simulink model "sim_2_3_matlab2024"  (R2024b)
settings: Solver=ode4  StartTime=0.0  StopTime=T_SIM  FixedStep=1e-3  RelTol=1e-3
values from neighbouring files (symbols this model uses):
  kf = 10    [EX_opt_2_leo.m]    (also in part2.m = 1; script_2_motion_planning.m)
  ki = 14    [EX_opt_2_leo.m]    (also in part2.m = 10; script_2_motion_planning.m = 4.5)
  qf = [1; 1; pi/2]    [EX_opt_2_leo.m]    (also in part2.m = [xf;yf;thetaf]; script_2_motion_planning.m)
  qi = [-1; -1; pi/2]    [EX_opt_2_leo.m]    (also in part2.m = [xi;yi;thetai]; script_2_motion_planning.m)
  Ta = 1    [fcn.m]    (also in part2.m = 2)
  Tc = 2    [fcn.m]    (also in part2.m = 3)
settings Model: Creator=alber  LastModifiedBy=loren
settings RTWCC: GPUComputeCapability=3.5

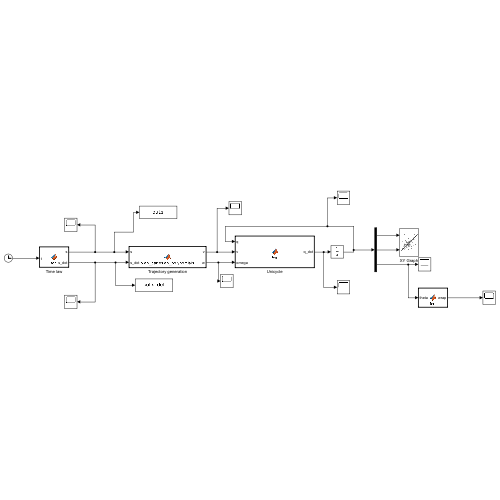
[thumbnail: Simulink's stored preview of the top-level diagram]
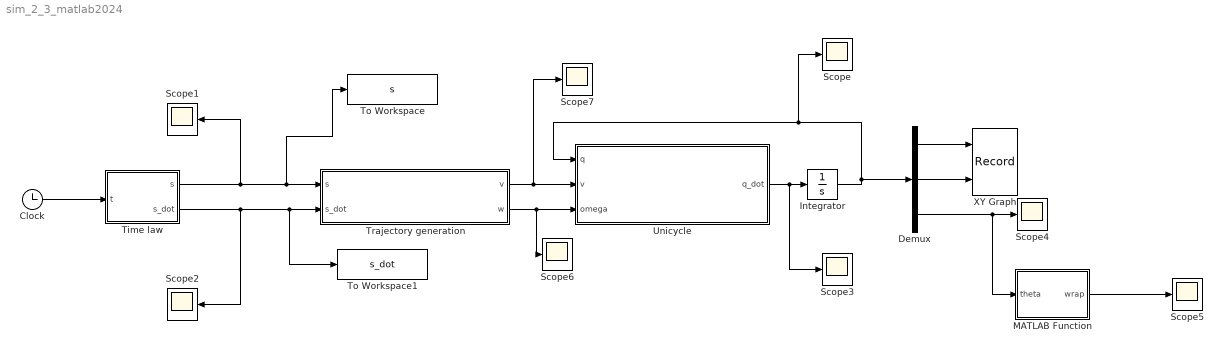
== system sim_2_3_matlab2024 ==
  Clock : Clock
  Demux : Demux  Outputs=3
  Integrator : Integrator  InitialCondition=qi
  MATLAB Function : MATLAB Function  TreatAsAtomicUnit=on
  Scope{,1..7} (8 alike) : Scope
  Time law : MATLAB Function  TreatAsAtomicUnit=on
  To Workspace : ToWorkspace  VariableName=s  SaveFormat=Timeseries  SampleTime=-1
  To Workspace1 : ToWorkspace  VariableName=s_dot  SaveFormat=Timeseries  SampleTime=-1
  Trajectory generation : MATLAB Function  TreatAsAtomicUnit=on
  Unicycle : MATLAB Function  TreatAsAtomicUnit=on
  XY Graph : Record  FileSettingsInternal="{\"entries\":[{\"content\":{\"excelSettings\":{\"content\":{},\"type\":\"Streamout.ExcelSettings\"}},\"type\":\"Streamout.FileSettingStorage\",\"uuid\":\"\"}],\"packageUris\":[\"http:\\/\\/schema.mathworks.com\\/mf0\\/streamout_blocks\\/R2020a\"],\"version\":\"1.0\"}"  Layout=[1 1]  SignalsInternal="{\"entries\":[{\"content\":{\"signals\":[{\"content\":{\"blockPath\":[],\"dimensions\":[1,1],\"domain\":\"\",\"lineColor\":\"#a2142f\",\"plots\":[ 1 ],\"port\":1,\"sid\":[\"\"],\"signalID\":1,\"signalName\":\"Demux:1\"},\"type\":\"RecordBlkView.Signal\",\"uuid\":\"\"},{\"content\":{\"blockPath\":[],\"dimensions\":[1,1],\"domain\":\"\",\"lineColor\":\"#139fff\",\"plots\":[ 1 ],\"port\":2,\"sid\":[\"\"],\"signalID\":2,\"signalName\":\"Demux:2\"},\"type\":\"RecordBlkView.Signal\",\"uuid\":\"\"}]},\"type\":\"RecordBlkView.InputSignals\",\"uuid\":\"\"}],\"packageUris\":[\"http:\\/\\/schema.mathworks.com\\/mf0\\/streamout_blocks\\/R2020a\"],\"version\":\"1.0\"}"  VisualizationBindings="{\"xyplotplugin\":{\"info\":[{\"series\":[{\"bindingParametersList\":[{\"parameter\":\"X-Axis\",\"signalID\":1,\"signalName\":\"Demux:1\"},{\"parameter\":\"Y-Axis\",\"signalID\":2,\"signalName\":\"Demux:2\"}],\"seriesID\":0}],\"subplotID\":1}]}}"  CompatibilityTag=XY
  wires:
  Clock/1 -> Time law/1(t)
  Time law/1(s) -> Scope1/1, To Workspace/1, Trajectory generation/1(s)
  Time law/2(s_dot) -> Scope2/1, To Workspace1/1, Trajectory generation/2(s_dot)
  Trajectory generation/1(v) -> Scope7/1, Unicycle/2(v)
  Trajectory generation/2(w) -> Scope6/1, Unicycle/3(omega)
  Unicycle/1(q_dot) -> Scope3/1, Integrator/1
  Demux/1 -> XY Graph/1
  Integrator/1 -> Scope/1, Unicycle/1(q), Demux/1
  MATLAB Function/1(wrap) -> Scope5/1
  Demux/2 -> XY Graph/2
  Demux/3 -> MATLAB Function/1(theta), Scope4/1

== matlab function sim_2_3_matlab2024/Trajectory generation ==
  data: s input; s_dot input; qi parameter; qf parameter; v output; w output; ki parameter; kf parameter
function [v, w] = plan_cartesian_polynomials(s, s_dot, qi, qf, ki, kf)
    % CUBIC POLYNOMIALS
    
    % Validity check for Simulink (fixed-size output)
    if ki * kf < 0
        v = 0; 
        w = 0;
        return;
    end
    
    % Extract initial and final states
    xi = qi(1); yi = qi(2); thetai = qi(3);
    xf = qf(1); yf = qf(2); thetaf = qf(3);
    
    % Compute coefficients a, b
    a = [xf, xi, kf*cos(thetaf)-3*xf, ki*cos(thetai)+3*xi ];
    b = [yf, yi, kf*sin(thetaf)-3*yf, ki*sin(thetai)+3*yi ];
    
    % Compute geometric derivatives
    % N.B. In Simulink 's' is a scalar at the current time step
    x_s_dot = 3*a(1)*s^2 - a(2)*(3*s^2 - 6*s + 3) + a(3)*(3*s^2 - 2*s) + a(4)*(3*s^2 - 4*s + 1);
    y_s_dot = 3*b(1)*s^2 - b(2)*(3*s^2 - 6*s + 3) + b(3)*(3*s^2 - 2*s) + b(4)*(3*s^2 - 4*s + 1);
    
    x_s_ddot = 6*a(1)*s - a(2)*(6*s - 6) + a(3)*(6*s - 2) + a(4)*(6*s - 4);
    y_s_ddot = 6*b(1)*s - b(2)*(6*s - 6) + b(3)*(6*s - 2) + b(4)*(6*s - 4);
    
    % Geometric inputs (with zero-division protection)
    v_tilde = sqrt(x_s_dot^2 + y_s_dot^2);
    
    % Adding 1e-6 prevents division by zero errors when the robot is stationary
    omega_tilde = (x_s_dot * y_s_ddot - y_s_dot * x_s_ddot) / (x_s_dot^2 + y_s_dot^2 + 1e-6);
    
    % Convert to real time inputs
    v = v_tilde * s_dot;
    w = omega_tilde * s_dot;
end

== matlab function sim_2_3_matlab2024/Time law ==
  data: t input; s output; s_dot output; Ta parameter; Tc parameter
function [s, s_dot] = fcn(t, Ta, Tc)

T1 = Ta;
T2 = Ta + Tc;
T3 = 2*Ta + Tc;

vc = 1/(Ta+Tc);
acc = vc/Ta;


% velocità
if t < T1
    s = 0.5*acc*t^2;
    s_dot = acc*t;

elseif t < T2
    s = 0.5*acc*Ta^2 + vc*(t - Ta);
    s_dot = vc;

elseif t < T3
    s = 0.5*acc*Ta^2 + vc*Tc + vc*(t - Ta - Tc)- 0.5*acc*(t - Ta - Tc)^2;
    s_dot = vc - acc*(t - Ta - Tc);

else
    s = 1;
    s_dot = 0;
end

== matlab function sim_2_3_matlab2024/Unicycle ==
  data: q_dot output; q input; v input; omega input
function q_dot = fcn(q, v, omega)
%write the unicycle model
q_dot= zeros(3,1);

q_dot(1) = v*cos(q(3));
q_dot(2) = v*sin(q(3));
q_dot(3) = omega;

== matlab function sim_2_3_matlab2024/MATLAB Function ==
  data: theta input; wrap output
function wrap = fcn(theta)

wrap = mod(theta+pi,2*pi)-pi ;
